simulink model "SMDM_Practica1"  (R2022b)
settings: Solver=VariableStepAuto  StartTime=0.0  StopTime=10.0  MaxStep=.00001  RelTol=1e-3
values from neighbouring files (symbols this model uses):
  g = 9.81    [CondicionesInicialesDoblePendulo.m]
  l1 = 0.3    [CondicionesInicialesDoblePendulo.m]
  l2 = 0.25    [CondicionesInicialesDoblePendulo.m]
  m1 = 0.2    [CondicionesInicialesDoblePendulo.m]
  m2 = 0.1    [CondicionesInicialesDoblePendulo.m]
settings Model: Creator=perez  LastModifiedBy=mluser

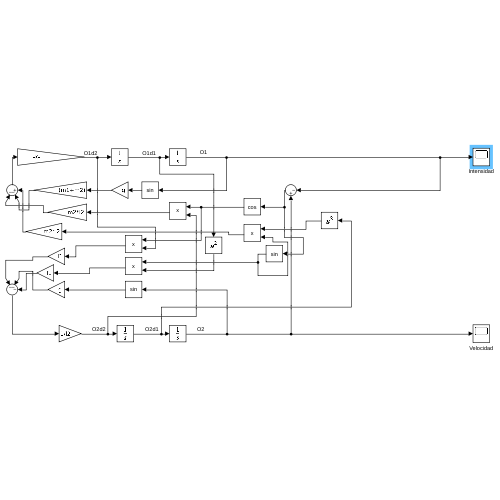
[thumbnail: Simulink's stored preview of the top-level diagram]
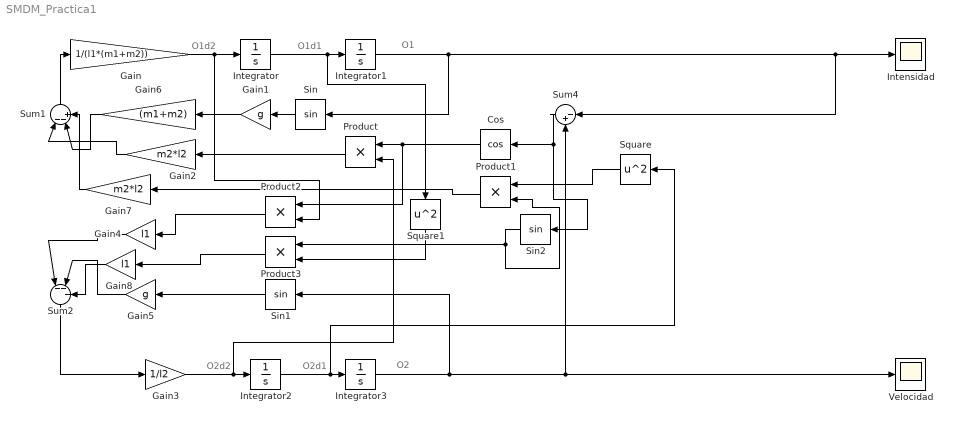
== system SMDM_Practica1 ==
  note: O2
  note: O2d1
  note: O2d2
  note: O1
  note: O1d1
  note: O1d2
  Cos : Trigonometry  Operator=cos
  Gain : Gain  Gain=1/(l1*(m1+m2))
  Gain1 : Gain  Gain=g
  Gain2 : Gain  Gain=m2*l2
  Gain3 : Gain  Gain=1/l2
  Gain4 : Gain  Gain=l1
  Gain5 : Gain  Gain=g
  Gain6 : Gain  Gain=(m1+m2)
  Gain7 : Gain  Gain=m2*l2
  Gain8 : Gain  Gain=l1
  Integrator : Integrator
  Integrator1 : Integrator
  Integrator2 : Integrator
  Integrator3 : Integrator  InitialCondition=(35*pi)/180
  Intensidad : Scope
  Product{,1..3} (4 alike) : Product
  Sin : Trigonometry
  Sin1 : Trigonometry
  Sin2 : Trigonometry
  Square : Math  Operator=square
  Square1 : Math  Operator=square
  Sum1 : Sum  Inputs=|--+
  Sum2 : Sum  Inputs=|---
  Sum4 : Sum  Inputs=|-+
  Velocidad : Scope
  wires:
  Gain/1 -> Product2/2, Integrator/1
  Integrator/1 -> Square1/1, Integrator1/1
  Sum1/1 -> Gain/1
  Gain1/1 -> Gain6/1
  Sin/1 -> Gain1/1
  Gain2/1 -> Sum1/1
  Product1/1 -> Gain7/1
  Product/1 -> Gain2/1
  Integrator3/1 -> Sin1/1, Sum4/2, Velocidad/1
  Integrator2/1 -> Square/1, Integrator3/1
  Gain3/1 -> Integrator2/1, Product/2
  Sum2/1 -> Gain3/1
  Gain5/1 -> Sum2/2
  Gain4/1 -> Sum2/1
  Sin1/1 -> Gain5/1
  Square/1 -> Product1/1
  Sum4/1 -> Sin2/1, Cos/1
  Sin2/1 -> Product1/2, Product3/1
  Square1/1 -> Product3/2
  Integrator1/1 -> Sin/1, Intensidad/1, Sum4/1
  Product3/1 -> Gain8/1
  Product2/1 -> Gain4/1
  Gain6/1 -> Sum1/2
  Cos/1 -> Product2/1, Product/1
  Gain7/1 -> Sum1/3
  Gain8/1 -> Sum2/3
